simulink model "Comp_TestBed1"  (R2019b)
settings: Solver=FixedStepDiscrete  StartTime=0.0  StopTime=inf  FixedStep=1  RelTol=1e-3  EnableMultiTasking=on
undefined symbols (not defined in the file): MWS, stripchar_TMATS
libraries: Lib_Turbo_Compressor_TMATS x1
settings Model: Creator=jwchapm2  LastModifiedBy=bhisma
settings DataIOCC: LimitDataPoints=on  SaveFormat=Array  ReturnWorkspaceOutputs=off
settings OptimizationCC: ExpressionDepthLimit=2147483647  LifeSpan=inf
settings DebuggingCC: UnderspecifiedInitializationDetection=Classic  MergeDetectMultiDrivingBlocksExec=none  SolverPrmCheckMsg=warning  StateNameClashWarn=warning  SFUnexpectedBacktrackingDiag=warning  SFNoUnconditionalDefaultTransitionDiag=warning  SFExecutionAtInitializationDiag=none  ArithmeticOperatorsInVariantConditions=warning
settings HardwareCC: ProdBitPerPointer=32  ProdBitPerSizeT=32  ProdBitPerPtrDiffT=32  ProdLargestAtomicFloat=None  ProdIntDivRoundTo=Undefined  ProdEndianess=Unspecified  ProdWordSize=32  ProdHWDeviceType=32-bit Generic
settings ModelReferenceCC: PropagateSignalLabelsOutOfModel=off
settings SFSimCC: SimUseLocalCustomCode=off  CustomCodeUndefinedFunction=UseInterfaceOnly
settings RTWCC: RTWUseLocalCustomCode=off
settings CodeAppCC: StateflowObjectComments=on
settings GRTTargetCC: TargetLangStandard=C89/C90 (ANSI)  GeneratePreprocessorConditionals=Disable all
settings ConfigComp: CovMetricSettings=dw  CovHtmlReporting=on  CovSaveCumulativeToWorkspaceVar=on  CovSaveSingleToWorkspaceVar=on  CovExternalEMLEnable=off

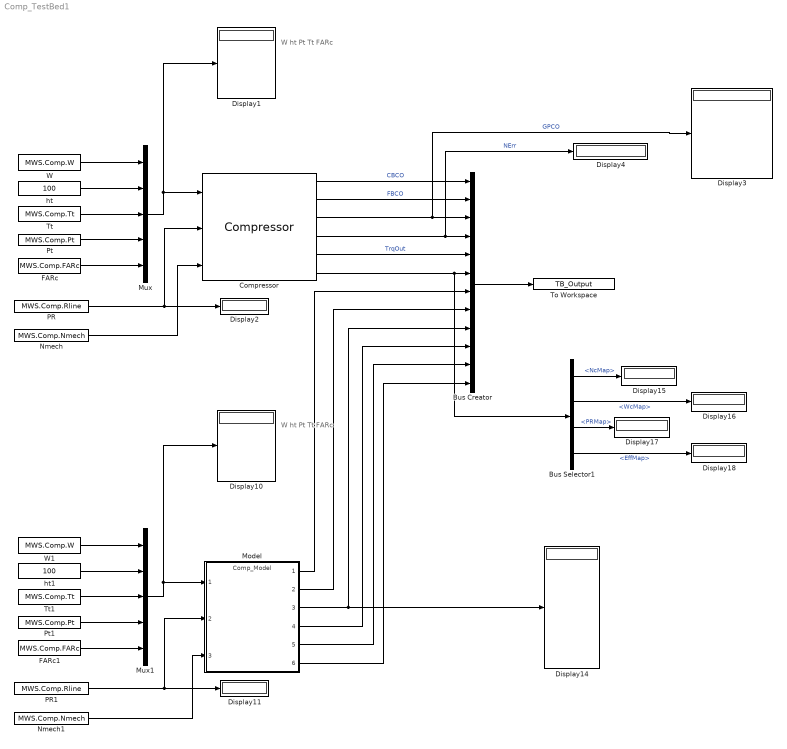
== system Comp_TestBed1 ==
  note: W
      | ht
      | Pt
      | Tt
      | FARc
  note: W
      | ht
      | Pt
      | Tt
      | FARc
  Bus Selector1 : BusSelector  OutputSignals=NcMap,WcMap,PRMap,EffMap
  Bus Creator : BusCreator  Inputs=12
  Compressor : Lib_Turbo_Compressor_TMATS/Compressor  X_C_RlineVec_M=MWS.Comp.RlineVec  Z_C_AlphaVec_M=1  Y_C_Map_NcVec_M=MWS.Comp.NcVec  T_C_Map_WcArray_M=MWS.Comp.WcArray  T_C_Map_PRArray_M=MWS.Comp.PRArray  T_C_Map_EffArray_M=MWS.Comp.EffArray  s_C_Nc_M=MWS.Comp.s_Nc  s_C_Wc_M=MWS.Comp.s_Wc  s_C_PR_M=MWS.Comp.s_PR  s_C_Eff_M=MWS.Comp.s_eff  SL_M=off  Scale_M=none  CBLDEN_M=on  C_CBD_M=MWS.Comp.CBD  C_CBFht_M=MWS.Comp.CBFht  C_CBFPt_M=MWS.Comp.CBFPt  FBLDEN_M=on  C_FBD_M=MWS.Comp.FBD  C_BFht_M=MWS.Comp.FBht  C_BFPt_M=MWS.Comp.FBPt  DefSMEn_M=off  SRline_M=1  X_C_Map_WcSurgeVec_M=MWS.Comp.WcSurgeVec  T_C_Map_PRSurgeVec_M=MWS.Comp.PRSugeVec  iDesign_M=2  NcDes_M=10000  EffDes_M=0.95  PRDes_M=20  RlineDes_M=2  FVar_M=strcat('iDes_',stripchar_TMATS(gcb),'.bin')  BlkNm_M=double(gcb)  HP_M=off
  Display{1..4,10..11,14..18} (11 alike) : Display
  FARc : Constant  Value=MWS.Comp.FARc
  FARc1 : Constant  Value=MWS.Comp.FARc
  Model : ModelReference  ModelNameDialog=Comp_Model.slx  SimulationMode=Normal  ModelReferenceVersion=1.7
  Mux : Mux  Inputs=5
  Mux1 : Mux  Inputs=5
  Nmech : Constant  Value=MWS.Comp.Nmech
  Nmech1 : Constant  Value=MWS.Comp.Nmech
  PR : Constant  Value=MWS.Comp.Rline
  PR1 : Constant  Value=MWS.Comp.Rline
  Pt : Constant  Value=MWS.Comp.Pt
  Pt1 : Constant  Value=MWS.Comp.Pt
  To Workspace : ToWorkspace  VariableName=TB_Output  SampleTime=-1
  Tt : Constant  Value=MWS.Comp.Tt
  Tt1 : Constant  Value=MWS.Comp.Tt
  W : Constant  Value=MWS.Comp.W
  W1 : Constant  Value=MWS.Comp.W
  ht : Constant  Value=100
  ht1 : Constant  Value=100
  wires:
  PR/1 -> Compressor/2, Display2/1
  W/1 -> Mux/1
  FARc/1 -> Mux/5
  Tt/1 -> Mux/3
  Pt/1 -> Mux/4
  Mux/1 -> Compressor/1, Display1/1
  Compressor/3 -> Display3/1, Bus Creator/3  "GPCO"
  Compressor/4 -> Display4/1, Bus Creator/4  "NErr"
  Compressor/5 -> Bus Creator/5  "TrqOut"
  Compressor/6 -> Bus Selector1/1, Bus Creator/6
  Bus Creator/1 -> To Workspace/1
  ht/1 -> Mux/2
  Nmech/1 -> Compressor/3
  Compressor/2 -> Bus Creator/2  "FBCO"
  Compressor/1 -> Bus Creator/1  "CBCO"
  PR1/1 -> Model/2, Display11/1
  W1/1 -> Mux1/1
  FARc1/1 -> Mux1/5
  Tt1/1 -> Mux1/3
  Pt1/1 -> Mux1/4
  Mux1/1 -> Model/1, Display10/1
  ht1/1 -> Mux1/2
  Bus Selector1/1 -> Display15/1  "<NcMap>"
  Bus Selector1/2 -> Display16/1  "<WcMap>"
  Bus Selector1/3 -> Display17/1  "<PRMap>"
  Bus Selector1/4 -> Display18/1  "<EffMap>"
  Model/5 -> Bus Creator/11
  Model/6 -> Bus Creator/12
  Nmech1/1 -> Model/3
  Model/1 -> Bus Creator/7
  Model/2 -> Bus Creator/8
  Model/3 -> Display14/1, Bus Creator/9
  Model/4 -> Bus Creator/10
